simulink model "z2"  (R2017b)
settings: Solver=VariableStepAuto  StartTime=0.0  StopTime=1  RelTol=1e-3
settings Model: Creator=Mahe  LastModifiedBy=Mahe

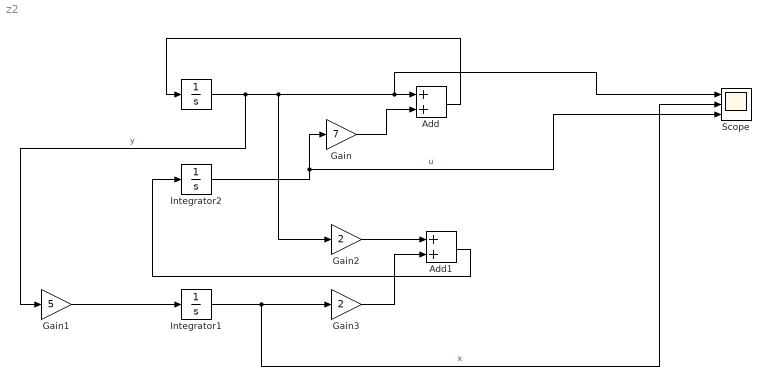
== system z2 ==
  " " : Integrator  InitialCondition=1
  Add : Sum
  Add1 : Sum
  Gain : Gain  Gain=7
  Gain1 : Gain  Gain=5
  Gain2 : Gain  Gain=2
  Gain3 : Gain  Gain=2
  Integrator1 : Integrator  InitialCondition=2
  Integrator2 : Integrator
  Scope : Scope  NumInputPorts=3
  wires:
  " "/1 -> Gain1/1, Gain2/1, Scope/1, Add/1  "y"
  Integrator1/1 -> Scope/2, Gain3/1  "x"
  Integrator2/1 -> Scope/3, Gain/1  "u"
  Gain/1 -> Add/2
  Add/1 -> " "/1
  Gain1/1 -> Integrator1/1
  Gain2/1 -> Add1/1
  Gain3/1 -> Add1/2
  Add1/1 -> Integrator2/1
